simulink model "Quad2DSimulinkController"  (R2023a)
settings: Solver=VariableStepAuto  StartTime=0.0  StopTime=10.0  RelTol=1e-3
values from neighbouring files (symbols this model uses):
  params =     [Quad2D_constants.mat]
undefined symbols (not defined in the file or in its folder): b_phi, b_y, b_z, init_phi, init_y, init_z, Kd, Kdt, Ki, Kp, Kpt, phi_des, z_des
settings Model: Creator=m260477  LastModifiedBy=m260477

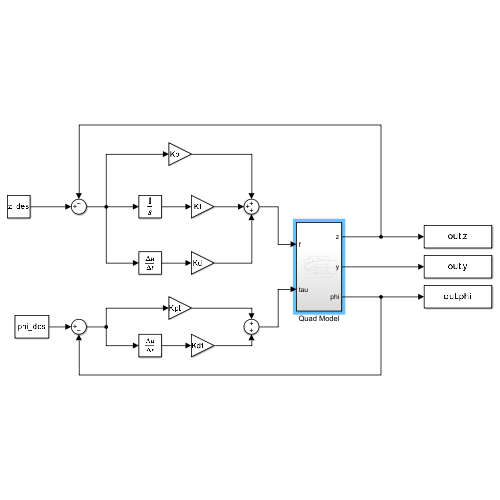
[thumbnail: Simulink's stored preview of the top-level diagram]
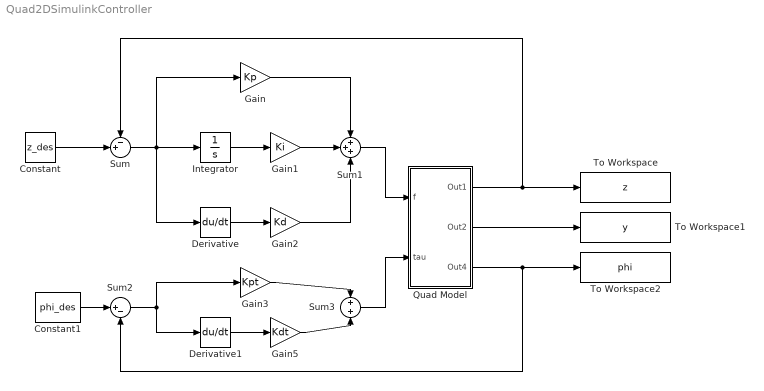
== system Quad2DSimulinkController ==
  Constant : Constant  Value=z_des
  Constant1 : Constant  Value=phi_des
  Derivative : Derivative
  Derivative1 : Derivative
  Gain : Gain  Gain=Kp
  Gain1 : Gain  Gain=Ki
  Gain2 : Gain  Gain=Kd
  Gain3 : Gain  Gain=Kpt
  Gain5 : Gain  Gain=Kdt
  Integrator : Integrator
  Quad Model : Subsystem
  Sum : Sum  Inputs=-+|
  Sum1 : Sum  Inputs=+++
  Sum2 : Sum  Inputs=|+-
  Sum3 : Sum
  To Workspace : ToWorkspace  VariableName=z  SaveFormat=Timeseries  SampleTime=-1
  To Workspace1 : ToWorkspace  VariableName=y  SaveFormat=Timeseries  SampleTime=-1
  To Workspace2 : ToWorkspace  VariableName=phi  SaveFormat=Timeseries  SampleTime=-1
  wires:
  Quad Model/1(Out1) -> Sum/1, To Workspace/1
  Quad Model/3(Out4) -> Sum2/2, To Workspace2/1
  Quad Model/2(Out2) -> To Workspace1/1
  Constant/1 -> Sum/2
  Sum1/1 -> Quad Model/1(f)
  Sum/1 -> Derivative/1, Integrator/1, Gain/1
  Gain/1 -> Sum1/1
  Gain1/1 -> Sum1/2
  Integrator/1 -> Gain1/1
  Gain2/1 -> Sum1/3
  Derivative/1 -> Gain2/1
  Gain3/1 -> Sum3/1
  Derivative1/1 -> Gain5/1
  Sum2/1 -> Derivative1/1, Gain3/1
  Gain5/1 -> Sum3/2
  Sum3/1 -> Quad Model/2(tau)
  Constant1/1 -> Sum2/1

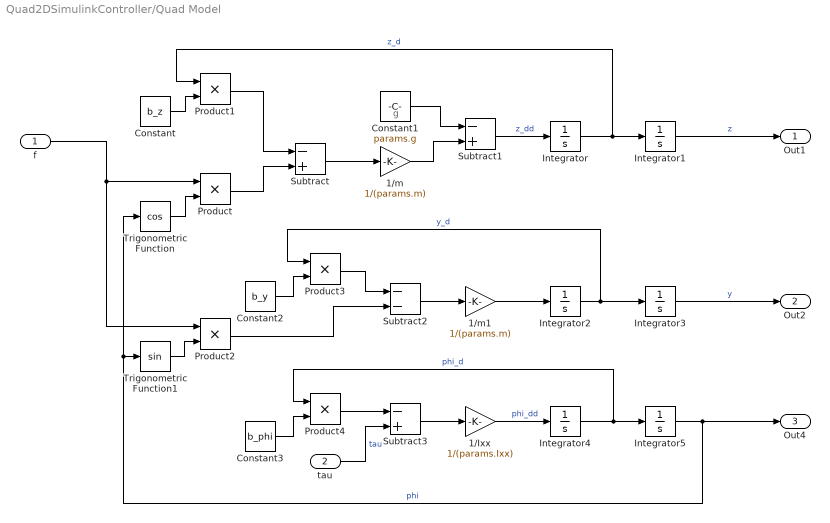
== system Quad2DSimulinkController/Quad Model ==
  note: g
  f : Inport
  tau : Inport  Port=2
  1/Ixx : Gain  Gain=1/(params.Ixx)
  1/m : Gain  Gain=1/(params.m)
  1/m1 : Gain  Gain=1/(params.m)
  Constant : Constant  Value=b_z
  Constant1 : Constant  Value=params.g
  Constant2 : Constant  Value=b_y
  Constant3 : Constant  Value=b_phi
  Integrator : Integrator
  Integrator1 : Integrator  InitialCondition=init_z
  Integrator2 : Integrator
  Integrator3 : Integrator  InitialCondition=init_y
  Integrator4 : Integrator
  Integrator5 : Integrator  InitialCondition=init_phi
  Product{,1..4} (5 alike) : Product
  Subtract : Sum  Inputs=-+
  Subtract1 : Sum  Inputs=-+
  Subtract2 : Sum  Inputs=--
  Subtract3 : Sum  Inputs=-+
  Trigonometric Function : Trigonometry  Operator=cos
  Trigonometric Function1 : Trigonometry
  Out1 : Outport
  Out2 : Outport  Port=2
  Out4 : Outport  Port=3
  wires:
  f/1 -> Product2/1, Product/1
  Subtract2/1 -> 1/m1/1
  Integrator1/1 -> Out1/1  "z"
  Integrator3/1 -> Out2/1  "y"
  Trigonometric Function/1 -> Product/2
  Integrator4/1 -> Product4/1, Integrator5/1  "phi_d"
  Integrator/1 -> Product1/1, Integrator1/1  "z_d"
  Constant/1 -> Product1/2
  Integrator2/1 -> Product3/1, Integrator3/1  "y_d"
  Constant3/1 -> Product4/2
  Product2/1 -> Subtract2/2
  Subtract1/1 -> Integrator/1  "z_dd"
  Constant2/1 -> Product3/2
  Product1/1 -> Subtract/1
  Product/1 -> Subtract/2
  Subtract3/1 -> 1/Ixx/1
  1/m/1 -> Subtract1/2
  1/Ixx/1 -> Integrator4/1  "phi_dd"
  Trigonometric Function1/1 -> Product2/2
  Constant1/1 -> Subtract1/1
  Integrator5/1 -> Out4/1, Trigonometric Function/1, Trigonometric Function1/1  "phi"
  tau/1 -> Subtract3/2  "tau"
  Product3/1 -> Subtract2/1
  1/m1/1 -> Integrator2/1
  Subtract/1 -> 1/m/1
  Product4/1 -> Subtract3/1
